simulink model "sm_forklift"  (R2021b)
settings: Solver=ode15s  StartTime=0.0  StopTime=53  MaxStep=1e-2  RelTol=1e-3  AbsTol=1e-3  EnableMultiTasking=on
model workspace: external: MATLAB File sm_forklift_parameters.m (data not in the file)
values from neighbouring files (symbols this model uses):
  g = 9.8    [sm_forklift_parameters.m]
undefined symbols (not defined in the file or in its folder): backRest, box, bump, chassis, fork, infPlane, main_mast, pulley, smiData, tire, top_mast, wheel, X, Y, Z
libraries: sm_lib x1413, nesl_utility x83, fl_lib x23, sm_backhoe_lib x6, SignalEditorBlockLib x1
(part 1 of 24)
settings Model: Creator=The MathWorks, Inc.  LastModifiedBy=The MathWorks, Inc.
settings SolverCC: AlgebraicLoopSolver=TrustRegion  SolverResetMethod=Robust
settings DataIOCC: LimitDataPoints=on  MaxDataPoints=10000  SaveTime=off  ReturnWorkspaceOutputs=off  SignalLoggingName=logsout_sm_forklift
settings OptimizationCC: LifeSpan=inf
settings DebuggingCC: AllowSymbolicDim=off  SFUnexpectedBacktrackingDiag=warning  SFNoUnconditionalDefaultTransitionDiag=warning  SFExecutionAtInitializationDiag=none  SFMachineParentedDataDiag=warning  ArithmeticOperatorsInVariantConditions=warning
settings SFSimCC: SimUseLocalCustomCode=off  CustomCodeUndefinedFunction=UseInterfaceOnly
settings RTWCC: RTWUseLocalCustomCode=off
settings CodeAppCC: StateflowObjectComments=on
settings GRTTargetCC: TargetLangStandard=C89/C90 (ANSI)
settings ConfigComp: CovMetricSettings=dw  CovSaveCumulativeToWorkspaceVar=on  CovSaveSingleToWorkspaceVar=on  CovExternalEMLEnable=off  CovSFcnEnable=off
settings SimscapeCC: SimscapeLogType=all  SimscapeLogSimulationStatistics=on  SimscapeLogName=simlog_sm_forklift  SimscapeLogLimitData=off  SimscapeLogDataHistory=10000
settings ExplorerConfigSet: InternalSimMechanicsExplorerSettings="<ExplorerConfiguration><canonicalview>planar_xy</canonicalview><AnimationSetting><BasePlaybackSpeed>1.0</BasePlaybackSpeed><PlaybackSpeedFactor>1.0</PlaybackSpeedFactor></AnimationSetting><TilePanel><TileInfo><Tiles Columns=\"1\" Count=\"2\" Rows=\"2\"><Column Weight=\"1\"/><Row Weight=\"0.6146\"/><Row Weight=\"0.3854\"/><Tile Height=\"1\" Width=\"1\" X=\"0\" Y=\"0\"/><Tile Height=\"1\" Width=\"1\" X=\"0\" Y=\"1\"/></Tiles></TileInfo><SceneInfo><SceneViewer><BGColor><R>0.800000011920928955</R><G>0.800000011920928955</G><B>0.800000011920928955</B></BGColor><Camera><DoPerspective>off</DoPerspective><Position><X>11.638287171197641</X><Y>5.89738784125214455</Y><Z>17.4286796258549366</Z></Position><Center><X>-3.00760539627548606</X><Y>1.55892249661538851</Y><Z>-1.63716110182111563</Z></Center><Up><X>-0.112390428536962572</X><Y>0.984091290920061201</Y><Z>-0.137596230720777618</Z></Up><ViewLimDist>1</ViewLimDist><YLim>4.35483527407086335</YLim><XLim>8.63886021848203711</XLim></Camera></SceneViewer><SceneViewer><BGColor><R>0.800000011920928955</R><G>0.800000011920928955</G><B>0.800000011920928955</B></BGColor><Camera><DoPerspective>off</DoPerspective><Position><X>-3.41673014646160489</X><Y>1.85826032602236757</Y><Z>21.8368627928964365</Z></Position><Center><X>-3.41673014646160489</X><Y>1.85826032602236757</Y><Z>-0.499999020020844398</Z></Center><Up><X>0</X><Y>1</Y><Z>0</Z></Up><ViewLimDist>1</ViewLimDist><YLim>3.43755894328755307</YLim><XLim>10.9285261519500061</XLim></Camera></SceneViewer></SceneInfo></TilePanel><MechEditorPanel><Cameras><Camera><Id>Camera1</Id><Value><Name>Camera1</Name><NativeCamera><PositionTrackingFeature>Forklift.Chassis.Cage.Frame2</PositionTrackingFeature><CenterTrackingFeature>Forklift.Forks.Pulley_Mechanism.PR</CenterTrackingFeature><UpVectorTrackingFeature>Forklift.Forks.Pulley_Mechanism.PR</UpVectorTrackingFeature><CenterTrackingOrigin>on</CenterTrackingOrigin><UpVectorTrackingDirection>+Y</UpVectorTrackingDirection></NativeCamera></Value></Camera></Cameras><GfxPanelCameraMap/><VideoCreator><PlaybackSpeedRatio>1.0</PlaybackSpeedRatio><FrameRate>60</FrameRate><VideoFormat>Motion JPEG AVI</VideoFormat><FrameSize>auto</FrameSize></VideoCreator></MechEditorPanel></ExplorerConfiguration>"

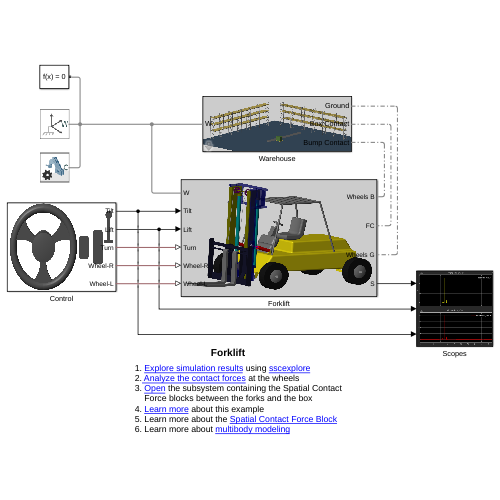
[thumbnail: Simulink's stored preview of the top-level diagram]
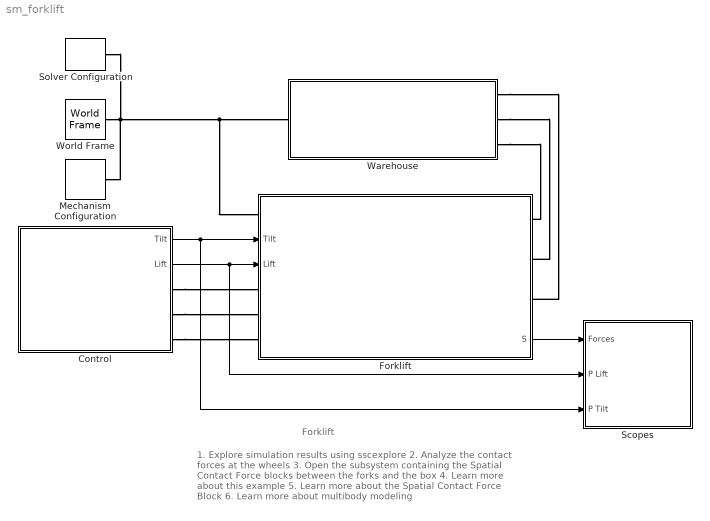
== system sm_forklift ==
  note: Forklift
  note: 1. Explore simulation results using sscexplore
      | 2. Analyze the contact forces at the wheels
      | 3. Open the subsystem containing the Spatial Contact
      | Force blocks between the forks and the box
      | 4. Learn more about this example
      | 5. Learn more about the Spatial Contact Force Block
      | 6. Learn more about multibody modeling
  Control : Subsystem
      mask Display:
      | image(fullfile(matlabroot,'toolbox','physmod','sm','smdemos',...
      |     'forklift','images','Driver_Inputs_IMAGE.png'));
  Forklift : Subsystem
      settings: PortSchema="{\"entries\":[{\"content\":{\"sides\":[{\"content\":{\"connectorIds\":[\"LConn1\",\"In1\",\"In2\",\"LConn2\",\"LConn3\",\"LConn4\"]},\"type\":\"ConnectorPlacement.EquallySpacedRectSide\",\"uuid\":\"b605c5d1-71b3-497b-b8b2-9d4274492848\"},{\"content\":{\"connectorIds\":[\"RConn1\",\"RConn2\",\"RConn3\",\"Out1\"],\"side\":\"RIGHT\"},\"type\":\"ConnectorPlacement.EquallySpacedRectSide\",\"uuid\":\"4a069455-70db-4f9b-8903-361922cdc27d\"},{\"content\":{\"connectorIds\":[],\"side\":\"TOP\"},\"type\":\"ConnectorPlacement.EquallySpacedRectSide\",\"uuid\":\"486f5f9e-cca7-41e2-8d21-59ab35260d28\"},{\"content\":{\"connectorIds\":[],\"side\":\"HIDDEN\"},\"type\":\"ConnectorPlacement.EquallySpacedRectSide\",\"uuid\":\"5ec2742c-19c2-4db8-b2a4-ecb60e15e59a\"}]},\"type\":\"ConnectorPlacement.EquallySpacedConnector\",\"uuid\":\"96ed48fc-1f8b-4fcb-b494-f6977a368fb7\"}],\"packageUris\":[\"http://schema.mathworks.com/mf0/Connector/R2020b\"],\"version\":\"1.0\"}"
      mask Display:
      | image(fullfile(matlabroot,'toolbox','physmod','sm','smdemos',...
      |     'forklift','images','Forklift.png'));
  Mechanism Configuration : sm_lib/Utilities/Mechanism Configuration  UniformGravity=Constant  GravityVector=[0 -g 0]  GravityUnits=m/s^2  LinearizationDelta=0.001  JointModeTransitionNonlinearIterations=2
  Scopes : Subsystem
      mask Display:
      | image(fullfile(matlabroot,'toolbox','physmod','sm','smdemos',...
      |     'forklift','images','scope.png'));
  Solver Configuration : nesl_utility/Solver Configuration  PhysicalDomain=network_engine_domain  SubClassName=solver  LeftPortType=input  RightPortType=generic  Tones=[]  Harmonics=[]  SimulateNoise=off  Profile=off  UseLocalSampling=off  EnableSwitchedLinearOptims=on  FrequencyDomain=off  UseCCode=off  RelTol=0.001  AbsTol=1e-06  MinStep=1e-09  ToWorkspace=off  RevertToSquareIcSolve=off  NumHomotopyIterations=100  PhasorMode=off  PhasorModeNumHarmonics=1  DoDC=off  ResidualTolerance=1e-09  UseLocalSolver=off  LocalSolverChoice=NE_BACKWARD_EULER_ADVANCER  LocalSolverSampleTime=0.001  DoFixedCost=off  MaxNonlinIter=3  MaxModeIter=2  ComputeImpulses=off  ImpulseIterations=1  LinearAlgebra=Sparse  EquationFormulation=NE_TIME_EF  DelaysMemoryBudget=1024  AutomaticFiltering=on  FilteringTimeConstant=0.001  PartitionStorageMethod=AS_NEEDED  PartitionMemoryBudget=1024  PartitionMethod=FAST
      settings: SourceProductBaseCode=PW,SS
  Warehouse : Subsystem  mask{infWidth=infPlane.width, infHeight=infPlane.height, infColor=infPlane.color, bRadius=bump.radius, bLength=bump.length, bColor=bump.color, bpDensity=box.base.density, bpColor=box.base.color, boxDimensions=box.dimensions, boxMass=box.mass, boxColor=box.color}
      mask prompts: infWidth "Width (m)"; infHeight "Height (m)"; infColor "Color"; bRadius "Radius (m)"; bLength "Length (m)"; bColor "Color"; bpDensity "Base Palet Density (kg/m^3)"; bpColor "Base Palet Color"; boxDimensions "Box Dimentions (m)"; boxMass "Box Mass (kg)"; boxColor "Box Color"
      mask DialogControl TabInfPlane Prompt: Infinite Plane
      mask DialogControl TabBump Prompt: Bump
      mask DialogControl TabLiftBox Prompt: Lifting Box
      mask Display:
      | image(fullfile(matlabroot,'toolbox','physmod','sm','smdemos',...
      |     'forklift','images','Warehouse.png'));
  World Frame : sm_lib/Frames and Transforms/World Frame
  wires:
  Control/1(Tilt) -> Scopes/3(P Tilt), Forklift/1(Tilt)
  Control/2(Lift) -> Scopes/2(P Lift), Forklift/2(Lift)
  Forklift/1(S) -> Scopes/1(Forces)
  connections:
  Solver Configuration/RConn1 -- Mechanism Configuration/RConn1 -- Forklift/LConn1 -- Warehouse/LConn1 -- World Frame/RConn1
  Warehouse/RConn3 -- Forklift/RConn1
  Warehouse/RConn2 -- Forklift/RConn2
  Warehouse/RConn1 -- Forklift/RConn3
  Control/RConn1 -- Forklift/LConn2
  Control/RConn2 -- Forklift/LConn3
  Control/RConn3 -- Forklift/LConn4

== system sm_forklift/Control ==
  Gain : Gain  Gain=5000
  Gain2 : Gain  Gain=4000
  Gain7 : Gain  Gain=0.25
  Gain8 : Gain  Gain=20
  PS Gain : fl_lib/Physical Signals/Functions/PS Gain  gain=-1
  Signal Editor : SignalEditorBlockLib/Signal Editor  FileName=Control_signals.mat  ActiveScenario=Scenario  ActiveSignal=Wheel  IsBus=off  OutputBusObjectStr=Bus: BusObject  SampleTime=0  ZeroCross=off  OutputAfterFinalValue=Holding final value  Unit=inherit  PreserveSignalName=on
  Simulink-PS Converter2 : nesl_utility/Simulink-PS Converter  PhysicalDomain=network_engine_domain  SubClassName=ps_input  LeftPortType=input  RightPortType=output  PseudoPeriodic=off  Frequencies=[]  NoiseDistribution=none  NoiseParameters=[]  Unit=1  AffineConversion=off  FilteringAndDerivatives=filter  SimscapeFilterOrder=2  InputFilterTimeConstant=0.01  UdotUserProvided=1
      settings: SourceProductBaseCode=PW,SS
  Simulink-PS Converter5 : nesl_utility/Simulink-PS Converter  PhysicalDomain=network_engine_domain  SubClassName=ps_input  LeftPortType=input  RightPortType=output  PseudoPeriodic=off  Frequencies=[]  NoiseDistribution=none  NoiseParameters=[]  Unit=1  AffineConversion=off  FilteringAndDerivatives=filter  SimscapeFilterOrder=2  InputFilterTimeConstant=0.01  UdotUserProvided=1
      settings: SourceProductBaseCode=PW,SS
  Turn : PMIOPort  Side=Right
  Wheel-R : PMIOPort  Port=2  Side=Right
  Wheel-L : PMIOPort  Port=3  Side=Right
  Tilt : Outport
  Lift : Outport  Port=2
  wires:
  Gain/1 -> Lift/1
  Gain8/1 -> Simulink-PS Converter2/1
  Gain7/1 -> Simulink-PS Converter5/1
  Gain2/1 -> Tilt/1
  Signal Editor/1 -> Gain2/1
  Signal Editor/2 -> Gain/1
  Signal Editor/3 -> Gain7/1
  Signal Editor/4 -> Gain8/1
  connections:
  PS Gain/RConn1 -- Wheel-R/RConn1
  Simulink-PS Converter5/RConn1 -- Turn/RConn1
  Simulink-PS Converter2/RConn1 -- PS Gain/LConn1 -- Wheel-L/RConn1

== system sm_forklift/Forklift ==
  Tilt : Inport
  Lift : Inport  Port=2
  6-DOF Joint : sm_lib/Joints/6-DOF Joint  JointMode=Normal  SenseConstraintForce=off  SenseConstraintForceX=off  SenseConstraintForceY=off  SenseConstraintForceZ=off  SenseConstraintTorque=off  SenseConstraintTorqueX=off  SenseConstraintTorqueY=off  SenseConstraintTorqueZ=off  SenseTotalForce=off  SenseTotalForceX=off  SenseTotalForceY=off  SenseTotalForceZ=off  SenseTotalTorque=off  SenseTotalTorqueX=off  SenseTotalTorqueY=off  SenseTotalTorqueZ=off  CompositeWrenchDir=FollowerOnBase  CompositeWrenchFrame=BaseFrame  PxEquilibriumPosition=0  PxEquilibriumPositionUnits=m  PxSpringStiffness=0  PxSpringStiffnessUnits=N/m  PxDampingCoefficient=0  PxDampingCoefficientUnits=N/(m/s)  PxTorqueActuationMode=NoTorque  PxMotionActuationMode=ComputedMotion  PxSensePosition=off  PxSenseVelocity=off  PxSenseAcceleration=off  PxSenseTorqueForce=off  PxSenseLowerLimitTorqueForce=off  PxSenseUpperLimitTorqueForce=off  PxLowerLimitSpecify=off  PxLowerLimitBound=-1  PxLowerLimitBoundUnits=m  PxLowerLimitStiffness=1e6  PxLowerLimitStiffnessUnits=N/m  PxLowerLimitDamping=1e3  PxLowerLimitDampingUnits=N/(m/s)  PxLowerLimitTransitionRegionWidth=1e-4  PxLowerLimitTransitionRegionWidthUnits=m  PxUpperLimitSpecify=off  PxUpperLimitBound=1  PxUpperLimitBoundUnits=m  PxUpperLimitStiffness=1e6  PxUpperLimitStiffnessUnits=N/m  PxUpperLimitDamping=1e3  PxUpperLimitDampingUnits=N/(m/s)  PxUpperLimitTransitionRegionWidth=1e-4  PxUpperLimitTransitionRegionWidthUnits=m  PxPositionTargetSpecify=off  PxPositionTargetPriority=High  PxPositionTargetValue=0  PxPositionTargetValueUnits=m  PxVelocityTargetSpecify=off  PxVelocityTargetPriority=High  PxVelocityTargetValue=0  PxVelocityTargetValueUnits=m/s  PyEquilibriumPosition=0  PyEquilibriumPositionUnits=m  PySpringStiffness=0  PySpringStiffnessUnits=N/m  PyDampingCoefficient=0  PyDampingCoefficientUnits=N/(m/s)  PyTorqueActuationMode=NoTorque  PyMotionActuationMode=ComputedMotion  PySensePosition=off  PySenseVelocity=off  PySenseAcceleration=off  PySenseTorqueForce=off  PySenseLowerLimitTorqueForce=off  PySenseUpperLimitTorqueForce=off  PyLowerLimitSpecify=off  PyLowerLimitBound=-1  PyLowerLimitBoundUnits=m  PyLowerLimitStiffness=1e6  PyLowerLimitStiffnessUnits=N/m  PyLowerLimitDamping=1e3  PyLowerLimitDampingUnits=N/(m/s)  PyLowerLimitTransitionRegionWidth=1e-4  PyLowerLimitTransitionRegionWidthUnits=m  PyUpperLimitSpecify=off  PyUpperLimitBound=1  PyUpperLimitBoundUnits=m  PyUpperLimitStiffness=1e6  PyUpperLimitStiffnessUnits=N/m  PyUpperLimitDamping=1e3  PyUpperLimitDampingUnits=N/(m/s)  PyUpperLimitTransitionRegionWidth=1e-4  PyUpperLimitTransitionRegionWidthUnits=m  PyPositionTargetSpecify=off  PyPositionTargetPriority=High  PyPositionTargetValue=0  PyPositionTargetValueUnits=m  PyVelocityTargetSpecify=off  PyVelocityTargetPriority=High  PyVelocityTargetValue=0  PyVelocityTargetValueUnits=m/s  PzEquilibriumPosition=0  PzEquilibriumPositionUnits=m  PzSpringStiffness=0  PzSpringStiffnessUnits=N/m  PzDampingCoefficient=0  PzDampingCoefficientUnits=N/(m/s)  PzTorqueActuationMode=NoTorque  PzMotionActuationMode=ComputedMotion  PzSensePosition=off  PzSenseVelocity=off  PzSenseAcceleration=off  PzSenseTorqueForce=off  PzSenseLowerLimitTorqueForce=off  PzSenseUpperLimitTorqueForce=off  PzLowerLimitSpecify=off  PzLowerLimitBound=-1  PzLowerLimitBoundUnits=m  PzLowerLimitStiffness=1e6  PzLowerLimitStiffnessUnits=N/m  PzLowerLimitDamping=1e3  PzLowerLimitDampingUnits=N/(m/s)  PzLowerLimitTransitionRegionWidth=1e-4  PzLowerLimitTransitionRegionWidthUnits=m  PzUpperLimitSpecify=off  PzUpperLimitBound=1  PzUpperLimitBoundUnits=m  PzUpperLimitStiffness=1e6  PzUpperLimitStiffnessUnits=N/m  PzUpperLimitDamping=1e3  PzUpperLimitDampingUnits=N/(m/s)  PzUpperLimitTransitionRegionWidth=1e-4  PzUpperLimitTransitionRegionWidthUnits=m  PzPositionTargetSpecify=off  PzPositionTargetPriority=High  PzPositionTargetValue=0  PzPositionTargetValueUnits=m  PzVelocityTargetSpecify=off  PzVelocityTargetPriority=High  PzVelocityTargetValue=0  PzVelocityTargetValueUnits=m/s  SphDefPosRotationMethod=None  SphDefPosRotationAngleUnits=deg  SphDefPosRotationStandardAxis=+Z  SphDefPosRotationAngle=0.0  SphDefPosRotationArbitraryAxis=[0 0 1]  SphDefPosFollAlignAxisA=+X  SphDefPosBaseAlignAxisA=+Y  SphDefPosFollAlignAxisB=+Y  SphDefPosBaseAlignAxisB=+Z  SphDefPosRotationSequenceAxes=FollowerAxes  SphDefPosRotationSequence=XYX  SphDefPosRotationSequenceAngles=[0 0 0]  SphDefPosRotationSequenceAnglesUnits=deg  SphDefPosRotationMatrix=[1 0 0; 0 1 0; 0 0 1]  SphEqPosRotationMethod=None  SphEqPosRotationAngleUnits=deg  SphEqPosRotationStandardAxis=+Z  SphEqPosRotationAngle=0.0  SphEqPosRotationArbitraryAxis=[0 0 1]  SphEqPosFollAlignAxisA=+X  SphEqPosBaseAlignAxisA=+Y  SphEqPosFollAlignAxisB=+Y  SphEqPosBaseAlignAxisB=+Z  SphEqPosRotationSequenceAxes=FollowerAxes  SphEqPosRotationSequence=XYX  SphEqPosRotationSequenceAngles=[0 0 0]  SphEqPosRotationSequenceAnglesUnits=deg  SphEqPosRotationMatrix=[1 0 0; 0 1 0; 0 0 1]  SphSpringStiffness=0  SphSpringStiffnessUnits=N*m/deg  SphDampingCoefficient=0  SphDampingCoefficientUnits=N*m/(deg/s)  SphActuateTorqueX=off  SphActuateTorqueY=off  SphActuateTorqueZ=off  SphActuateTorque=off  SphTorqueActuationMode=NoTorque  SphMotionActuationMode=ComputedMotion  SphActuationFrame=BaseFrame  SphSensePosition=off  SphSenseVelocityX=off  SphSenseVelocityY=off  SphSenseVelocityZ=off  SphSenseVelocity=off  SphSenseAccelerationX=off  SphSenseAccelerationY=off  SphSenseAccelerationZ=off  SphSenseAcceleration=off  SphSenseTorqueX=off  SphSenseTorqueY=off  SphSenseTorqueZ=off  SphSenseTorqueForce=off  SphSenseLowerLimitTorqueMag=off  SphSenseUpperLimitTorqueMag=off  SphSensingFrame=BaseFrame  SphLowerLimitSpecify=off  SphLowerLimitBound=15  SphLowerLimitBoundUnits=deg  SphLowerLimitStiffness=1e4  SphLowerLimitStiffnessUnits=N*m/deg  SphLowerLimitDamping=10  SphLowerLimitDampingUnits=N*m/(deg/s)  SphLowerLimitTransitionRegionWidth=0.1  SphLowerLimitTransitionRegionWidthUnits=deg  SphUpperLimitSpecify=off  SphUpperLimitBound=45  SphUpperLimitBoundUnits=deg  SphUpperLimitStiffness=1e4  SphUpperLimitStiffnessUnits=N*m/deg  SphUpperLimitDamping=10  SphUpperLimitDampingUnits=N*m/(deg/s)  SphUpperLimitTransitionRegionWidth=0.1  SphUpperLimitTransitionRegionWidthUnits=deg  SphPositionTargetRotationMethod=None  SphPositionTargetRotationAngleUnits=deg  SphPositionTargetRotationStandardAxis=+Z  SphPositionTargetRotationAngle=0.0  SphPositionTargetRotationArbitraryAxis=[0 0 1]  SphPositionTargetFollAlignAxisA=+X  SphPositionTargetBaseAlignAxisA=+Y  SphPositionTargetFollAlignAxisB=+Y  SphPositionTargetBaseAlignAxisB=+Z  SphPositionTargetRotationSequenceAxes=FollowerAxes  SphPositionTargetRotationSequence=XYX  SphPositionTargetRotationSequenceAngles=[0 0 0]  SphPositionTargetRotationSequenceAnglesUnits=deg  SphPositionTargetRotationMatrix=[1 0 0; 0 1 0; 0 0 1]  SphPositionTargetSpecify=off  SphPositionTargetPriority=High  SphVelocityTargetValue=[0 0 0]  SphVelocityTargetValueUnits=deg/s  SphVelocityTargetSpecify=off  SphVelocityTargetPriority=High  SphVelocityTargetInFollowerFrame=on
  Bus Creator : BusCreator  Inputs=2
  Chassis : Subsystem  mask{m=chassis.weight, ChassisColor=chassis.color}
      mask prompts: m "Chassis Base Mass (kg)"; ChassisColor "Chassis Color"
      mask DialogControl ChassisInertia Prompt: Inertia
      mask DialogControl ChassisGraphic Prompt: Graphic
      mask Display:
      | image(fullfile(matlabroot,'toolbox','physmod','sm','smdemos',...
      |     'forklift','images','Chassis.png'));
  Forks : Subsystem  mask{pMass=pulley.mass, pColor=pulley.color, brMass=backRest.mass, brColor=backRest.color, fMass=fork.mass, fColor=fork.color, fStiffness=fork.contact.stiffness, fDamping=fork.contact.damping, fTransWidth=fork.contact.transitionRegion, fStatic=fork.contact.staticFriction, fDynamic=fork.contact.dynamicFriction, fCritical=fork.contact.criticalVelocity, pointVisible=off}
      mask prompts: pMass "Pulley Mass (kg)"; pColor "Pulley Color"; brMass "Back Rest Mass (kg)"; brColor "Back Rest Color"; fMass "Fork Mass (kg)"; fColor "Fork Color"; fStiffness "Contact Stiffness (N/m)"; fDamping "Contact Damping (N/(m/s))"; fTransWidth "Transition Region Width (m)"; fStatic "Static Friction"; fDynamic "Dynamic Friction"; fCritical "Critical Velocity (m/s)"; pointVisible "Make fork contact points visible"
      mask init:
      | if (pointVisible == 0)
      |     set_param('sm_forklift/Forklift/Forks/Fork Contacts/Point16',"GraphicType",'None');
      |     set_param('sm_forklift/Forklift/Forks/Fork Contacts/Point20',"GraphicType",'None');
      |     set_param('sm_forklift/Forklift/Forks/Fork Contacts/Point22',"GraphicType",'None');
      |     set_param('sm_forklift/Forklift/Forks/Fork Contacts/Point25',"GraphicType",'None');
      |     set_param('sm_forklift/Forklift/Forks/Fork Contacts/Point4',"GraphicType",'None');
      |     set_param('sm_forklift/Forklift/Forks/Fork Contacts/Point26',"GraphicType",'None');
      |     set_param('sm_forklift/Forklift/Forks/Fork Contacts/Point30',"GraphicType",'None');
      |     set_param('sm_forklift/Forklift/Forks/Fork Contacts/Point32',"GraphicType",'None');
      |     set_param('sm_forklift/Forklift/Forks/Fork Contacts/Point35',"GraphicType",'None');
      |     set_param('sm_forklift/Forklift/Forks/Fork Contacts/Point6',"GraphicType",'None');
      |     set_param('sm_forklift/Forklift/Forks/Fork Contacts/Point12',"GraphicType",'None');
      |     set_param('sm_forklift/Forklift/Forks/Fork Contacts/Point13',"GraphicType",'None');
      |     set_param('sm_forklift/Forklift/Forks/Fork Contacts/Point14',"GraphicType",'None');
      |     set_param('sm_forklift/Forklift/Forks/Fork Contacts/Point15',"GraphicType",'None');
      |     set_param('sm_forklift/Forklift/Forks/Fork Contacts/Point10',"GraphicType",'None');
      |     set_param('sm_forklift/Forklift/Forks/Fork Contacts/Point46',"GraphicType",'None');
      |     set_param('sm_forklift/Forklift/Forks/Fork Contacts/Point50',"GraphicType",'None');
      |     set_param('sm_forklift/Forklift/Forks/Fork Contacts/Point54',"GraphicType",'None');
      |     set_param('sm_forklift/Forklift/Forks/Fork Contacts/Point55',"GraphicType",'None');
      |     set_param('sm_forklift/Forklift/Forks/Fork Contacts/Point36',"GraphicType",'None');
      |     set_param('sm_forklift/Forklift/Forks/Fork Contacts/Point40',"GraphicType",'None');
      |     set_param('sm_forklift/Forklift/Forks/Fork Contacts/Point41',"GraphicType",'None');
      |     set_param('sm_forklift/Forklift/Forks/Fork Contacts/Point45',"GraphicType",'None');
      |     set_param('sm_forklift/Forklift/Forks/Fork Contacts/Point11',"GraphicType",'None');
      |     set_param('sm_forklift/Forklift/Forks/Fork Contacts/Point5',"GraphicType",'None');
      |     set_param('sm_forklift/Forklift/Forks/Fork Contacts/Point7',"GraphicType",'None');
      |     set_param('sm_forklift/Forklift/Forks/Fork Contacts/Point8',"GraphicType",'None');
      |     set_param('sm_forklift/Forklift/Forks/Fork Contacts/Point9',"GraphicType",'None');
      | else
      |     set_param('sm_forklift/Forklift/Forks/Fork Contacts/Point16',"GraphicType",'Marker');
      |     set_param('sm_forklift/Forklift/Forks/Fork Contacts/Point20',"GraphicType",'Marker');
      |     set_param('sm_forklift/Forklift/Forks/Fork Contacts/Point22',"GraphicType",'Marker');
      |     set_param('sm_forklift/Forklift/Forks/Fork Contacts/Point25',"GraphicType",'Marker');
      |     set_param('sm_forklift/Forklift/Forks/Fork Contacts/Point4',"GraphicType",'Marker');
      |     set_param('sm_forklift/Forklift/Forks/Fork Contacts/Point26',"GraphicType",'Marker');
      |     set_param('sm_forklift/Forklift/Forks/Fork Contacts/Point30',"GraphicType",'Marker');
      |     set_param('sm_forklift/Forklift/Forks/Fork Contacts/Point32',"GraphicType",'Marker');
      |     set_param('sm_forklift/Forklift/Forks/Fork Contacts/Point35',"GraphicType",'Marker');
      |     set_param('sm_forklift/Forklift/Forks/Fork Contacts/Point6',"GraphicType",'Marker');
      |     set_param('sm_forklift/Forklift/Forks/Fork Contacts/Point12',"GraphicType",'Marker');
      |     set_param('sm_forklift/Forklift/Forks/Fork Contacts/Point13',"GraphicType",'Marker');
      |     set_param('sm_forklift/Forklift/Forks/Fork Contacts/Point14',"GraphicType",'Marker');
      |     set_param('sm_forklift/Forklift/Forks/Fork Contacts/Point15',"GraphicType",'Marker');
      |     set_param('sm_forklift/Forklift/Forks/Fork Contacts/Point10',"GraphicType",'Marker');
      |     set_param('sm_forklift/Forklift/Forks/Fork Contacts/Point46',"GraphicType",'Marker');
      |     set_param('sm_forklift/Forklift/Forks/Fork Contacts/Point50',"GraphicType",'Marker');
      |     set_param('sm_forklift/Forklift/Forks/Fork Contacts/Point54',"GraphicType",'Marker');
      |     set_param('sm_forklift/Forklift/Forks/Fork Contacts/Point55',"GraphicType",'Marker');
      |     set_param('sm_forklift/Forklift/Forks/Fork Contacts/Point36',"GraphicType",'Marker');
      |     set_param('sm_forklift/Forklift/Forks/Fork Contacts/Point40',"GraphicType",'Marker');
      |     set_param('sm_forklift/Forklift/Forks/Fork Contacts/Point41',"GraphicType",'Marker');
      |     set_param('sm_forklift/Forklift/Forks/Fork Contacts/Point45',"GraphicType",'Marker');
      |     set_param('sm_forklift/Forklift/Forks/Fork Contacts/Point11',"GraphicType",'Marker');
      |     set_param('sm_forklift/Forklift/Forks/Fork Contacts/Point5',"GraphicType",'Marker');
      |     set_param('sm_forklift/Forklift/Forks/Fork Contacts/Point7',"GraphicType",'Marker');
      |     set_param('sm_forklift/Forklift/Forks/Fork Contacts/Point8',"GraphicType",'Marker');
      |     set_param('sm_forklift/Forklift/Forks/Fork Contacts/Point9',"GraphicType",'Marker');  
      | end
      settings: PortSchema="{\"entries\":[{\"content\":{\"sides\":[{\"content\":{\"connectorIds\":[\"LConn1\",\"LConn2\",\"LConn3\",\"LConn4\",\"LConn5\"]},\"type\":\"ConnectorPlacement.EquallySpacedRectSide\",\"uuid\":\"f89f8a38-021e-4541-8e29-613773e12899\"},{\"content\":{\"connectorIds\":[\"RConn1\",\"Out1\"],\"side\":\"RIGHT\"},\"type\":\"ConnectorPlacement.EquallySpacedRectSide\",\"uuid\":\"9e861d83-a9bf-4b00-b212-9617c64b8fa6\"},{\"content\":{\"connectorIds\":[],\"side\":\"TOP\"},\"type\":\"ConnectorPlacement.EquallySpacedRectSide\",\"uuid\":\"a9ae9b03-e52b-4809-8f23-580f29ab349c\"},{\"content\":{\"connectorIds\":[],\"side\":\"HIDDEN\"},\"type\":\"ConnectorPlacement.EquallySpacedRectSide\",\"uuid\":\"904f46d3-97de-456d-88f0-f4c445169ffa\"}]},\"type\":\"ConnectorPlacement.EquallySpacedConnector\",\"uuid\":\"2f7ec563-5437-47e3-ae24-442ff138a9a0\"}],\"packageUris\":[\"http://schema.mathworks.com/mf0/Connector/R2020b\"],\"version\":\"1.0\"}"
      mask DialogControl TabPulley Prompt: Pulleys
      mask DialogControl PulleyInertia Prompt: Inertia
      mask DialogControl PulleyGraphic Prompt: Graphic
      mask DialogControl TabBackRest Prompt: Back Rest
      mask DialogControl BackRestInertia Prompt: Inertia
      mask DialogControl BackRestGraphic Prompt: Graphic
      mask DialogControl TabFork Prompt: Fork
      mask DialogControl ForkInertia Prompt: Inertia
      mask DialogControl ForkGraphic Prompt: Graphic
      mask DialogControl ForkContacts Prompt: Fork Contacts
      mask Display:
      | image(fullfile(matlabroot,'toolbox','physmod','sm','smdemos',...
      |     'forklift','images','Forks.png'));
  Left Front Wheel : sm_lib/Joints/Revolute Joint  JointMode=Normal  SenseConstraintForce=off  SenseConstraintForceX=off  SenseConstraintForceY=off  SenseConstraintForceZ=off  SenseConstraintTorque=off  SenseConstraintTorqueX=off  SenseConstraintTorqueY=off  SenseConstraintTorqueZ=off  SenseTotalForce=off  SenseTotalForceX=off  SenseTotalForceY=off  SenseTotalForceZ=off  SenseTotalTorque=off  SenseTotalTorqueX=off  SenseTotalTorqueY=off  SenseTotalTorqueZ=off  CompositeWrenchDir=FollowerOnBase  CompositeWrenchFrame=BaseFrame  EquilibriumPosition=0  EquilibriumPositionUnits=deg  SpringStiffness=0  SpringStiffnessUnits=N*m/deg  DampingCoefficient=0  DampingCoefficientUnits=N*m/(deg/s)  TorqueActuationMode=ComputedTorque  MotionActuationMode=InputMotion  SensePosition=off  SenseVelocity=off  SenseAcceleration=off  SenseTorqueForce=off  SenseLowerLimitTorqueForce=off  SenseUpperLimitTorqueForce=off  LowerLimitSpecify=off  LowerLimitBound=-90  LowerLimitBoundUnits=deg  LowerLimitStiffness=1e4  LowerLimitStiffnessUnits=N*m/deg  LowerLimitDamping=10  LowerLimitDampingUnits=N*m/(deg/s)  LowerLimitTransitionRegionWidth=0.1  LowerLimitTransitionRegionWidthUnits=deg  UpperLimitSpecify=off  UpperLimitBound=90  UpperLimitBoundUnits=deg  UpperLimitStiffness=1e4  UpperLimitStiffnessUnits=N*m/deg  UpperLimitDamping=10  UpperLimitDampingUnits=N*m/(deg/s)  UpperLimitTransitionRegionWidth=0.1  UpperLimitTransitionRegionWidthUnits=deg  PositionTargetSpecify=off  PositionTargetPriority=High  PositionTargetValue=0  PositionTargetValueUnits=deg  VelocityTargetSpecify=off  VelocityTargetPriority=High  VelocityTargetValue=0  VelocityTargetValueUnits=deg/s
  Left Rear Wheel : sm_lib/Joints/Revolute Joint  JointMode=Normal  SenseConstraintForce=off  SenseConstraintForceX=off  SenseConstraintForceY=off  SenseConstraintForceZ=off  SenseConstraintTorque=off  SenseConstraintTorqueX=off  SenseConstraintTorqueY=off  SenseConstraintTorqueZ=off  SenseTotalForce=off  SenseTotalForceX=off  SenseTotalForceY=off  SenseTotalForceZ=off  SenseTotalTorque=off  SenseTotalTorqueX=off  SenseTotalTorqueY=off  SenseTotalTorqueZ=off  CompositeWrenchDir=FollowerOnBase  CompositeWrenchFrame=BaseFrame  EquilibriumPosition=0  EquilibriumPositionUnits=deg  SpringStiffness=0  SpringStiffnessUnits=N*m/deg  DampingCoefficient=0  DampingCoefficientUnits=N*m/(deg/s)  TorqueActuationMode=NoTorque  MotionActuationMode=ComputedMotion  SensePosition=off  SenseVelocity=off  SenseAcceleration=off  SenseTorqueForce=off  SenseLowerLimitTorqueForce=off  SenseUpperLimitTorqueForce=off  LowerLimitSpecify=off  LowerLimitBound=-90  LowerLimitBoundUnits=deg  LowerLimitStiffness=1e4  LowerLimitStiffnessUnits=N*m/deg  LowerLimitDamping=10  LowerLimitDampingUnits=N*m/(deg/s)  LowerLimitTransitionRegionWidth=0.1  LowerLimitTransitionRegionWidthUnits=deg  UpperLimitSpecify=off  UpperLimitBound=90  UpperLimitBoundUnits=deg  UpperLimitStiffness=1e4  UpperLimitStiffnessUnits=N*m/deg  UpperLimitDamping=10  UpperLimitDampingUnits=N*m/(deg/s)  UpperLimitTransitionRegionWidth=0.1  UpperLimitTransitionRegionWidthUnits=deg  PositionTargetSpecify=off  PositionTargetPriority=High  PositionTargetValue=0  PositionTargetValueUnits=deg  VelocityTargetSpecify=off  VelocityTargetPriority=High  VelocityTargetValue=0  VelocityTargetValueUnits=deg/s
  Masts : Subsystem
      settings: PortSchema="{\"entries\":[{\"content\":{\"sides\":[{\"content\":{\"connectorIds\":[\"In1\",\"In2\"]},\"type\":\"ConnectorPlacement.EquallySpacedRectSide\",\"uuid\":\"c11de26c-6c1c-4f27-ab79-7250c95e36e0\"},{\"content\":{\"connectorIds\":[\"RConn1\",\"RConn2\",\"RConn3\",\"RConn4\",\"RConn5\"],\"side\":\"RIGHT\"},\"type\":\"ConnectorPlacement.EquallySpacedRectSide\",\"uuid\":\"7023b709-a1b2-4247-bb57-7da3a4e272f4\"},{\"content\":{\"connectorIds\":[],\"side\":\"TOP\"},\"type\":\"ConnectorPlacement.EquallySpacedRectSide\",\"uuid\":\"60704e78-2733-42ec-9594-3c7d77e4de86\"},{\"content\":{\"connectorIds\":[\"RConn6\",\"RConn7\",\"RConn8\",\"RConn9\"],\"side\":\"BOTTOM\"},\"type\":\"ConnectorPlacement.EquallySpacedRectSide\",\"uuid\":\"590320fa-9bb4-45a1-bb01-92ca190eb04d\"},{\"content\":{\"connectorIds\":[],\"side\":\"HIDDEN\"},\"type\":\"ConnectorPlacement.EquallySpacedRectSide\",\"uuid\":\"da325ca6-01c3-45e6-b6eb-0c9b8ab20db2\"}]},\"type\":\"ConnectorPlacement.EquallySpacedConnector\",\"uuid\":\"2d73e1a7-b822-4218-bf29-ca24980a07fe\"}],\"packageUris\":[\"http://schema.mathworks.com/mf0/Connector/R2020b\"],\"version\":\"1.0\"}"
      mask Display:
      | image(fullfile(matlabroot,'toolbox','physmod','sm','smdemos',...
      |     'forklift','images','Masts.png'));
  Prismatic Joint Fork to Outer : sm_lib/Joints/Prismatic Joint  JointMode=Normal  SenseConstraintForce=off  SenseConstraintForceX=off  SenseConstraintForceY=off  SenseConstraintForceZ=off  SenseConstraintTorque=off  SenseConstraintTorqueX=off  SenseConstraintTorqueY=off  SenseConstraintTorqueZ=off  SenseTotalForce=off  SenseTotalForceX=off  SenseTotalForceY=off  SenseTotalForceZ=off  SenseTotalTorque=off  SenseTotalTorqueX=off  SenseTotalTorqueY=off  SenseTotalTorqueZ=off  CompositeWrenchDir=FollowerOnBase  CompositeWrenchFrame=BaseFrame  EquilibriumPosition=0  EquilibriumPositionUnits=m  SpringStiffness=0  SpringStiffnessUnits=N/m  DampingCoefficient=0  DampingCoefficientUnits=N/(m/s)  TorqueActuationMode=NoTorque  MotionActuationMode=ComputedMotion  SensePosition=off  SenseVelocity=off  SenseAcceleration=off  SenseTorqueForce=off  SenseLowerLimitTorqueForce=off  SenseUpperLimitTorqueForce=off  LowerLimitSpecify=on  LowerLimitBound=-1  LowerLimitBoundUnits=m  LowerLimitStiffness=1e6  LowerLimitStiffnessUnits=N/m  LowerLimitDamping=1e3  LowerLimitDampingUnits=N/(m/s)  LowerLimitTransitionRegionWidth=1e-4  LowerLimitTransitionRegionWidthUnits=m  UpperLimitSpecify=on  UpperLimitBound=0  UpperLimitBoundUnits=m  UpperLimitStiffness=1e6  UpperLimitStiffnessUnits=N/m  UpperLimitDamping=1e3  UpperLimitDampingUnits=N/(m/s)  UpperLimitTransitionRegionWidth=1e-4  UpperLimitTransitionRegionWidthUnits=m  PositionTargetSpecify=off  PositionTargetPriority=High  PositionTargetValue=0  PositionTargetValueUnits=m  VelocityTargetSpecify=off  VelocityTargetPriority=High  VelocityTargetValue=0  VelocityTargetValueUnits=m/s
  Right Front Wheel : sm_lib/Joints/Revolute Joint  JointMode=Normal  SenseConstraintForce=off  SenseConstraintForceX=off  SenseConstraintForceY=off  SenseConstraintForceZ=off  SenseConstraintTorque=off  SenseConstraintTorqueX=off  SenseConstraintTorqueY=off  SenseConstraintTorqueZ=off  SenseTotalForce=off  SenseTotalForceX=off  SenseTotalForceY=off  SenseTotalForceZ=off  SenseTotalTorque=off  SenseTotalTorqueX=off  SenseTotalTorqueY=off  SenseTotalTorqueZ=off  CompositeWrenchDir=FollowerOnBase  CompositeWrenchFrame=BaseFrame  EquilibriumPosition=0  EquilibriumPositionUnits=deg  SpringStiffness=0  SpringStiffnessUnits=N*m/deg  DampingCoefficient=0  DampingCoefficientUnits=N*m/(deg/s)  TorqueActuationMode=ComputedTorque  MotionActuationMode=InputMotion  SensePosition=off  SenseVelocity=off  SenseAcceleration=off  SenseTorqueForce=off  SenseLowerLimitTorqueForce=off  SenseUpperLimitTorqueForce=off  LowerLimitSpecify=off  LowerLimitBound=-90  LowerLimitBoundUnits=deg  LowerLimitStiffness=1e4  LowerLimitStiffnessUnits=N*m/deg  LowerLimitDamping=10  LowerLimitDampingUnits=N*m/(deg/s)  LowerLimitTransitionRegionWidth=0.1  LowerLimitTransitionRegionWidthUnits=deg  UpperLimitSpecify=off  UpperLimitBound=90  UpperLimitBoundUnits=deg  UpperLimitStiffness=1e4  UpperLimitStiffnessUnits=N*m/deg  UpperLimitDamping=10  UpperLimitDampingUnits=N*m/(deg/s)  UpperLimitTransitionRegionWidth=0.1  UpperLimitTransitionRegionWidthUnits=deg  PositionTargetSpecify=off  PositionTargetPriority=High  PositionTargetValue=0  PositionTargetValueUnits=deg  VelocityTargetSpecify=off  VelocityTargetPriority=High  VelocityTargetValue=0  VelocityTargetValueUnits=deg/s
  Right Rear Wheel : sm_lib/Joints/Revolute Joint  JointMode=Normal  SenseConstraintForce=off  SenseConstraintForceX=off  SenseConstraintForceY=off  SenseConstraintForceZ=off  SenseConstraintTorque=off  SenseConstraintTorqueX=off  SenseConstraintTorqueY=off  SenseConstraintTorqueZ=off  SenseTotalForce=off  SenseTotalForceX=off  SenseTotalForceY=off  SenseTotalForceZ=off  SenseTotalTorque=off  SenseTotalTorqueX=off  SenseTotalTorqueY=off  SenseTotalTorqueZ=off  CompositeWrenchDir=FollowerOnBase  CompositeWrenchFrame=BaseFrame  EquilibriumPosition=0  EquilibriumPositionUnits=deg  SpringStiffness=0  SpringStiffnessUnits=N*m/deg  DampingCoefficient=0  DampingCoefficientUnits=N*m/(deg/s)  TorqueActuationMode=NoTorque  MotionActuationMode=ComputedMotion  SensePosition=off  SenseVelocity=off  SenseAcceleration=off  SenseTorqueForce=off  SenseLowerLimitTorqueForce=off  SenseUpperLimitTorqueForce=off  LowerLimitSpecify=off  LowerLimitBound=-90  LowerLimitBoundUnits=deg  LowerLimitStiffness=1e4  LowerLimitStiffnessUnits=N*m/deg  LowerLimitDamping=10  LowerLimitDampingUnits=N*m/(deg/s)  LowerLimitTransitionRegionWidth=0.1  LowerLimitTransitionRegionWidthUnits=deg  UpperLimitSpecify=off  UpperLimitBound=90  UpperLimitBoundUnits=deg  UpperLimitStiffness=1e4  UpperLimitStiffnessUnits=N*m/deg  UpperLimitDamping=10  UpperLimitDampingUnits=N*m/(deg/s)  UpperLimitTransitionRegionWidth=0.1  UpperLimitTransitionRegionWidthUnits=deg  PositionTargetSpecify=off  PositionTargetPriority=High  PositionTargetValue=0  PositionTargetValueUnits=deg  VelocityTargetSpecify=off  VelocityTargetPriority=High  VelocityTargetValue=0  VelocityTargetValueUnits=deg/s
  Wheels : Subsystem  mask{wRadius=wheel.radius, wWidth=wheel.width, wAxle=wheel.axleRadius, wResolution=wheel.resolution, wDensity=wheel.density, wColor=wheel.color, TireRadius=tire.radius, TireDensity=tire.density, TireColor=tire.color, wStiffness=wheel.contact.stiffness, wDamping=wheel.contact.damping, wTransWidth=wheel.contact.transitionRegion, wStatic=wheel.contact.staticFriction, wDynamic=wheel.contact.dynamicFriction, wCritical=wheel.contact.criticalVelocity}
      mask prompts: wRadius "Radius (m)"; wWidth "Width (m)"; wAxle "Axle Radius (m)"; wResolution "Circle Resolution (pts/rev)"; wDensity "Wheel Density (kg/m^3)"; wColor "Color"; TireRadius "Radius (m)"; TireDensity "Density (kg/m^3)"; TireColor "Color"; wStiffness "Contact Stiffness (N/m)"; wDamping "Contact Damping (N/(m/s))"; wTransWidth "Transition Region Width (mm)"; wStatic "Static Friction"; wDynamic "Dynamic Friction"; wCritical "Critical Velocity (m/s)"
      settings: PortSchema="{\"entries\":[{\"content\":{\"sides\":[{\"content\":{\"connectorIds\":[\"LConn1\",\"LConn2\"]},\"type\":\"ConnectorPlacement.EquallySpacedRectSide\",\"uuid\":\"674a5221-c1b0-416a-ae59-2f7d63171317\"},{\"content\":{\"connectorIds\":[\"Out1\",\"RConn1\",\"RConn2\"],\"side\":\"RIGHT\"},\"type\":\"ConnectorPlacement.EquallySpacedRectSide\",\"uuid\":\"d242f688-68f2-44b4-8ad4-b3cdbde7b357\"},{\"content\":{\"connectorIds\":[\"LConn3\",\"LConn4\"],\"side\":\"TOP\"},\"type\":\"ConnectorPlacement.EquallySpacedRectSide\",\"uuid\":\"7630af07-5f56-4f50-9a9c-5d9b13470242\"},{\"content\":{\"connectorIds\":[],\"side\":\"HIDDEN\"},\"type\":\"ConnectorPlacement.EquallySpacedRectSide\",\"uuid\":\"41a5c749-e566-40b6-8bd4-889630ae8a96\"}]},\"type\":\"ConnectorPlacement.EquallySpacedConnector\",\"uuid\":\"7346caf9-6a4c-4ee7-acbb-0fac498f8199\"}],\"packageUris\":[\"http://schema.mathworks.com/mf0/Connector/R2020b\"],\"version\":\"1.0\"}"
      mask DialogControl TabWheel Prompt: Wheel
      mask DialogControl WheelGeometry Prompt: Geometry
      mask DialogControl WheelInertia Prompt: Inertia
      mask DialogControl WheelGraphic Prompt: Graphic
      mask DialogControl TabTire Prompt: Tire
      mask DialogControl TireGeometry Prompt: Geometry
      mask DialogControl TireInertia Prompt: Inertia
      mask DialogControl TireGraphic Prompt: Graphic
      mask DialogControl WheelContacts Prompt: Wheel Contacts
      mask Display:
      | image(fullfile(matlabroot,'toolbox','physmod','sm','smdemos',...
      |     'forklift','images','Wheels.png'));
  W : PMIOPort  Side=Left
  Turn : PMIOPort  Port=2  Side=Left
  Wheel-R : PMIOPort  Port=3  Side=Left
  Wheel-L : PMIOPort  Port=4  Side=Left
  Wheels B : PMIOPort  Port=5  Side=Right
  FC : PMIOPort  Port=6  Side=Right
  Wheels G : PMIOPort  Port=7  Side=Right
  S : Outport
  wires:
  Tilt/1 -> Masts/1(P Tilt)
  Lift/1 -> Masts/2(P Lift)
  Wheels/1(S) -> Bus Creator/2
  Forks/1(S) -> Bus Creator/1
  Bus Creator/1 -> S/1
  connections:
  Chassis/LConn1 -- 6-DOF Joint/RConn1
  Turn/RConn1 -- Chassis/LConn2
  Wheels/LConn4 -- Left Front Wheel/RConn1
  Right Front Wheel/RConn1 -- Wheels/LConn3
  Wheels/LConn2 -- Right Rear Wheel/RConn1
  Wheels/LConn1 -- Left Rear Wheel/RConn1
  Wheels B/RConn1 -- Wheels/RConn1
  Wheels G/RConn1 -- Wheels/RConn2
  Masts/RConn6 -- Chassis/RConn1
  Masts/RConn7 -- Chassis/RConn2
  Masts/RConn8 -- Chassis/RConn3
  Chassis/RConn4 -- Masts/RConn9
  Forks/LConn1 -- Prismatic Joint Fork to Outer/RConn1
  Masts/RConn2 -- Forks/LConn2
  Masts/RConn3 -- Forks/LConn3
  Forks/LConn4 -- Masts/RConn4
  Masts/RConn5 -- Forks/LConn5
  FC/RConn1 -- Forks/RConn1
  6-DOF Joint/LConn1 -- W/RConn1
  Wheel-R/RConn1 -- Right Front Wheel/LConn2
  Left Front Wheel/LConn1 -- Chassis/RConn5
  Wheel-L/RConn1 -- Left Front Wheel/LConn2
  Chassis/RConn6 -- Right Front Wheel/LConn1
  Left Rear Wheel/LConn1 -- Chassis/RConn8
  Right Rear Wheel/LConn1 -- Chassis/RConn7
  Prismatic Joint Fork to Outer/LConn1 -- Masts/RConn1

== system sm_forklift/Scopes ==
  Forces : Inport
  P Lift : Inport  Port=2
  P Tilt : Inport  Port=3
  Bus Selector : BusSelector  OutputSignals=signal2.NomalForce_WheelLF,signal2.FrictionalForce_WheelLF,signal2.NomalForce_WheelRF,signal2.FrictionalForce_WheelRF,signal2.NomalForce_WheelRR,signal2.FrictionalForce_WheelRR,signal2.NomalForce_WheelLR,signal2.FrictionalForce_WheelLR,signal1.ContactForceBetweenForks&Box
  Scope{1..4} (4 alike) : Scope  NumInputPorts=2
  Scope5 : Scope
  Scope6 : Scope
  Scope7 : Scope
  wires:
  Bus Selector/3 -> Scope2/1  "<NomalForce_WheelRF>"
  Bus Selector/8 -> Scope4/2  "<FrictionalForce_WheelLR>"
  Bus Selector/9 -> Scope5/1  "<ContactForceBetweenForks&Box>"
  Bus Selector/4 -> Scope2/2  "<FrictionalForce_WheelRF>"
  Bus Selector/5 -> Scope3/1  "<NomalForce_WheelRR>"
  Bus Selector/7 -> Scope4/1  "<NomalForce_WheelLR>"
  Bus Selector/6 -> Scope3/2  "<FrictionalForce_WheelRR>"
  P Lift/1 -> Scope6/1  "Hydraulic Lift Pressure"
  Bus Selector/1 -> Scope1/1  "<NomalForce_WheelLF>"
  Bus Selector/2 -> Scope1/2  "<FrictionalForce_WheelLF>"
  Forces/1 -> Bus Selector/1
  P Tilt/1 -> Scope7/1  "Hydraulic Tilt Pressure"
